simulink model "mrefrobotarm_modified_previous_y_previous_u_previous_ref_prepro"  (R2018b)
settings: Solver=FixedStepAuto  StartTime=0.0  StopTime=10  RelTol=1e-3  AbsTol=1e-6
undefined symbols (not defined in the file or in its folder): cc, options
libraries: neural x594, simulink x1
(part 12 of 22)

== system mrefrobotarm_modified_previous_y_previous_u_previous_ref_prepro/pre_0.00002/Layer 3/Delays 1 ==
  "p{3}" : Inport  PortDimensions=30
      mask Display: e = 0.06;c1 = [120 230 180]/255;c2 = ([120 230 180]+0)/(256+128);c3 = ([120 230 180]+128)/(256+128);patch([0 1 1 0],[0 0 1 1],c1);patch([0 1 1 1-e 1-e 0+e],[0 0 1 1-e 0+e 0+e],c2);patch([0 0 1 1-e 0+e 0+e],[0 1 1 1-e 1-e 0+e],c3);plot([0 1 1 0 0],[0 0 1 1 0]);
  mux : Mux  Inputs=1
      mask Display: e = 0.06;c1 = [120 150 230]/255;c2 = ([120 150 230]+0)/383;c3 = ([120 150 230]+128)/383;patch([0 1 1 0],[0 0 1 1],c1);patch([0 1 1 1-e 1-e 0+e],[0 0 1 1-e 0+e 0+e],c2);patch([0 0 1 1-e 0+e 0+e],[0 1 1 1-e 1-e 0+e],c3);plot([0 1 1 0 0],[0 0 1 1 0]);disp('Mux')
  "pd{3,2}" : Outport
      mask Display: e = 0.06;c1 = [120 230 180]/255;c2 = ([120 230 180]+0)/(256+128);c3 = ([120 230 180]+128)/(256+128);patch([0 1 1 0],[0 0 1 1],c1);patch([0 1 1 1-e 1-e 0+e],[0 0 1 1-e 0+e 0+e],c2);patch([0 0 1 1-e 0+e 0+e],[0 1 1 1-e 1-e 0+e],c3);plot([0 1 1 0 0],[0 0 1 1 0]);
  wires:
  "p{3}"/1 -> mux/1
  mux/1 -> "pd{3,2}"/1

== system mrefrobotarm_modified_previous_y_previous_u_previous_ref_prepro/pre_0.00002/Layer 3/LW{3,2} ==
  "ad{3,2}" : Inport  PortDimensions=30
      mask Display: e = 0.06;c1 = [120 230 180]/255;c2 = ([120 230 180]+0)/(256+128);c3 = ([120 230 180]+128)/(256+128);patch([0 1 1 0],[0 0 1 1],c1);patch([0 1 1 1-e 1-e 0+e],[0 0 1 1-e 0+e 0+e],c2);patch([0 0 1 1-e 0+e 0+e],[0 1 1 1-e 1-e 0+e],c3);plot([0 1 1 0 0],[0 0 1 1 0]);
  "IW{3,2}(1,:)'" : Constant  Value=[0.026357043524044672377915077277066302485764026641845703125;-0.51872721281168232554392716338043101131916046142578125;0.06788526676316682106904210058928583748638629913330078125;0.1504865458343480622005472469027154147624969482421875;0.2009539872745570165957218478069989942014217376708984375;-0.25736048987968518364510828178026713430881500244140625;0.4746746233954628468865166723844595253467559814453125;0.09619380315352972499187700350375962443649768829345703125;-0.39222775076773885860603741093655116856098175048828125;0.58814532203051161918239131409791298210620880126953125;-0.0090835429099451990564428882635183981619775295257568359375;0.02668635591032859910587404783655074425041675567626953125;-0.29710748430544153819710118114016950130462646484375;-0.30678250346949997862111558788456022739410400390625;-0.18096965580139234841539064291282556951045989990234375;-0.65963002624456257283469540197984315454959869384765625;0.483992188838884784818361595171154476702213287353515625;0.0026123351413663013949328917107095548999495804309844970703125;0.02009700292768311358226895890766172669827938079833984375;0.11671148285488382179142519134984468109905719757080078125;-0.134139518384796152528082302524126134812831878662109375;0.34435981653929437218408793341950513422489166259765625;0.151399461664854573239580304289120249450206756591796875;-0.429360650055773229727407169775688089430332183837890625;0.40448496021973412428707206345279701054096221923828125;0.255568865447091175813199015465215779840946197509765625;0.38427145101844495389542544216965325176715850830078125;-0.53491524948961555185888983032782562077045440673828125;0.2358667832365416161533033800878911279141902923583984375;-1.269425035749180974420369238941930234432220458984375]
      mask Display: e = 0.06;c1 = [120 150 230]/255;c2 = ([120 150 230]+0)/383;c3 = ([120 150 230]+128)/383;patch([0 1 1 0],[0 0 1 1],c1);patch([0 1 1 1-e 1-e 0+e],[0 0 1 1-e 0+e 0+e],c2);patch([0 0 1 1-e 0+e 0+e],[0 1 1 1-e 1-e 0+e],c3);plot([0 1 1 0 0],[0 0 1 1 0]);disp('weights');
  Mux : Mux  Inputs=1
      mask Display: e = 0.06;c1 = [120 150 230]/255;c2 = ([120 150 230]+0)/383;c3 = ([120 150 230]+128)/383;patch([0 1 1 0],[0 0 1 1],c1);patch([0 1 1 1-e 1-e 0+e],[0 0 1 1-e 0+e 0+e],c2);patch([0 0 1 1-e 0+e 0+e],[0 1 1 1-e 1-e 0+e],c3);plot([0 1 1 0 0],[0 0 1 1 0]);disp('Mux');
  dotprod1 : neural/Weight Functions/dotprod
  "lz{3,2}" : Outport
      mask Display: e = 0.06;c1 = [120 230 180]/255;c2 = ([120 230 180]+0)/(256+128);c3 = ([120 230 180]+128)/(256+128);patch([0 1 1 0],[0 0 1 1],c1);patch([0 1 1 1-e 1-e 0+e],[0 0 1 1-e 0+e 0+e],c2);patch([0 0 1 1-e 0+e 0+e],[0 1 1 1-e 1-e 0+e],c3);plot([0 1 1 0 0],[0 0 1 1 0]);
  wires:
  "IW{3,2}(1,:)'"/1 -> dotprod1/1
  "ad{3,2}"/1 -> dotprod1/2
  dotprod1/1 -> Mux/1
  Mux/1 -> "lz{3,2}"/1

== system mrefrobotarm_modified_previous_y_previous_u_previous_ref_prepro/pre_0.00003/Layer 1/Delays 1 ==
  "p{1}" : Inport  PortDimensions=10
      mask Display: e = 0.06;c1 = [120 230 180]/255;c2 = ([120 230 180]+0)/(256+128);c3 = ([120 230 180]+128)/(256+128);patch([0 1 1 0],[0 0 1 1],c1);patch([0 1 1 1-e 1-e 0+e],[0 0 1 1-e 0+e 0+e],c2);patch([0 0 1 1-e 0+e 0+e],[0 1 1 1-e 1-e 0+e],c3);plot([0 1 1 0 0],[0 0 1 1 0]);
  mux : Mux  Inputs=1
      mask Display: e = 0.06;c1 = [120 150 230]/255;c2 = ([120 150 230]+0)/383;c3 = ([120 150 230]+128)/383;patch([0 1 1 0],[0 0 1 1],c1);patch([0 1 1 1-e 1-e 0+e],[0 0 1 1-e 0+e 0+e],c2);patch([0 0 1 1-e 0+e 0+e],[0 1 1 1-e 1-e 0+e],c3);plot([0 1 1 0 0],[0 0 1 1 0]);disp('Mux')
  "pd{1,1}" : Outport
      mask Display: e = 0.06;c1 = [120 230 180]/255;c2 = ([120 230 180]+0)/(256+128);c3 = ([120 230 180]+128)/(256+128);patch([0 1 1 0],[0 0 1 1],c1);patch([0 1 1 1-e 1-e 0+e],[0 0 1 1-e 0+e 0+e],c2);patch([0 0 1 1-e 0+e 0+e],[0 1 1 1-e 1-e 0+e],c3);plot([0 1 1 0 0],[0 0 1 1 0]);
  wires:
  "p{1}"/1 -> mux/1
  mux/1 -> "pd{1,1}"/1

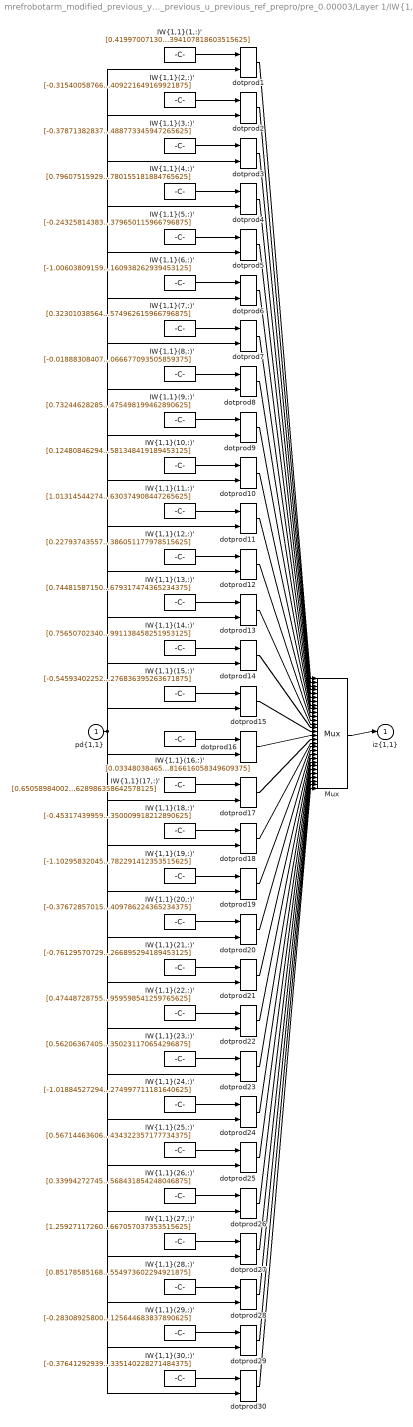
== system mrefrobotarm_modified_previous_y_previous_u_previous_ref_prepro/pre_0.00003/Layer 1/IW{1,1} ==
  "pd{1,1}" : Inport  PortDimensions=10
      mask Display: e = 0.06;c1 = [120 230 180]/255;c2 = ([120 230 180]+0)/(256+128);c3 = ([120 230 180]+128)/(256+128);patch([0 1 1 0],[0 0 1 1],c1);patch([0 1 1 1-e 1-e 0+e],[0 0 1 1-e 0+e 0+e],c2);patch([0 0 1 1-e 0+e 0+e],[0 1 1 1-e 1-e 0+e],c3);plot([0 1 1 0 0],[0 0 1 1 0]);
  "IW{1,1}(1,:)'" : Constant  Value=[0.419970071301938474572779114168952219188213348388671875;-0.8435648108302473691111345033277757465839385986328125;-0.1656764929854205037340619810493080876767635345458984375;-0.11639218277869724238460236165337846614420413970947265625;-1.0085904908462273166236400356865487992763519287109375;0.2870157504733672482188922003842890262603759765625;0.51428228640491180367888546243193559348583221435546875;0.54134778151221329967057727117207832634449005126953125;0.4535298805716763137496627678046934306621551513671875;-0.80929306256536348573860095712007023394107818603515625]
      mask Display: e = 0.06;c1 = [120 150 230]/255;c2 = ([120 150 230]+0)/383;c3 = ([120 150 230]+128)/383;patch([0 1 1 0],[0 0 1 1],c1);patch([0 1 1 1-e 1-e 0+e],[0 0 1 1-e 0+e 0+e],c2);patch([0 0 1 1-e 0+e 0+e],[0 1 1 1-e 1-e 0+e],c3);plot([0 1 1 0 0],[0 0 1 1 0]);disp('Weights');
  "IW{1,1}(10,:)'" : Constant  Value=[0.1248084629473502626950676130945794284343719482421875;0.5561546445854499420846650536986999213695526123046875;-0.000113541552609613440039115772606237442232668399810791015625;-1.267332618187496873218833570717833936214447021484375;1.324848031024380201614576435531489551067352294921875;0.435693687642321469954964641146943904459476470947265625;-0.8716286812435034558887991806841455399990081787109375;0.039256312878930797738430413801324903033673763275146484375;0.24291130218279122221503030232270248234272003173828125;0.579349644472149094553969916887581348419189453125]
      mask Display: e = 0.06;c1 = [120 150 230]/255;c2 = ([120 150 230]+0)/383;c3 = ([120 150 230]+128)/383;patch([0 1 1 0],[0 0 1 1],c1);patch([0 1 1 1-e 1-e 0+e],[0 0 1 1-e 0+e 0+e],c2);patch([0 0 1 1-e 0+e 0+e],[0 1 1 1-e 1-e 0+e],c3);plot([0 1 1 0 0],[0 0 1 1 0]);disp('Weights');
  "IW{1,1}(11,:)'" : Constant  Value=[1.013145442746719471216465535690076649188995361328125;0.99243177005728810957663199587841518223285675048828125;0.7891671128990978001382927686790935695171356201171875;0.99448519338468754913407110507250763475894927978515625;0.78513301503203092313043498506885953247547149658203125;1.039734908888301223583994215005077421665191650390625;0.0113187088607663612072062875313349650241434574127197265625;0.450506637373380869338035381588269956409931182861328125;0.463038284909750241791215330522391013801097869873046875;0.08865900952312423533019369870089576579630374908447265625]
      mask Display: e = 0.06;c1 = [120 150 230]/255;c2 = ([120 150 230]+0)/383;c3 = ([120 150 230]+128)/383;patch([0 1 1 0],[0 0 1 1],c1);patch([0 1 1 1-e 1-e 0+e],[0 0 1 1-e 0+e 0+e],c2);patch([0 0 1 1-e 0+e 0+e],[0 1 1 1-e 1-e 0+e],c3);plot([0 1 1 0 0],[0 0 1 1 0]);disp('Weights');
  "IW{1,1}(12,:)'" : Constant  Value=[0.2279374355718996325581571227303356863558292388916015625;-0.72859698297398123312262896433821879327297210693359375;0.47417467679467184549224612055695615708827972412109375;0.990640763171337201953292606049217283725738525390625;0.09802646157368609391991043366942903958261013031005859375;-0.1375834764035423207761965613826760090887546539306640625;0.94485525986767082695649833112838678061962127685546875;-0.089139203371477238047049240776686929166316986083984375;0.348785768332843748584792820111033506691455841064453125;-0.70331874474973388178256072933436371386051177978515625]
      mask Display: e = 0.06;c1 = [120 150 230]/255;c2 = ([120 150 230]+0)/383;c3 = ([120 150 230]+128)/383;patch([0 1 1 0],[0 0 1 1],c1);patch([0 1 1 1-e 1-e 0+e],[0 0 1 1-e 0+e 0+e],c2);patch([0 0 1 1-e 0+e 0+e],[0 1 1 1-e 1-e 0+e],c3);plot([0 1 1 0 0],[0 0 1 1 0]);disp('Weights');
  "IW{1,1}(13,:)'" : Constant  Value=[0.7448158715080184233414684058516286313533782958984375;-0.937709653184260805147687278804369270801544189453125;0.21308729556658556614223698488785885274410247802734375;0.89987770978577519276342400189605541527271270751953125;-0.5439743765683768828012034646235406398773193359375;1.540566291152452915724779813899658620357513427734375;-0.1376689897811968210650235278080799616873264312744140625;-0.228351277546065489776339063610066659748554229736328125;0.038462164544626441242680670029585598967969417572021484375;-0.57219919711055788891229667569859884679317474365234375]
      mask Display: e = 0.06;c1 = [120 150 230]/255;c2 = ([120 150 230]+0)/383;c3 = ([120 150 230]+128)/383;patch([0 1 1 0],[0 0 1 1],c1);patch([0 1 1 1-e 1-e 0+e],[0 0 1 1-e 0+e 0+e],c2);patch([0 0 1 1-e 0+e 0+e],[0 1 1 1-e 1-e 0+e],c3);plot([0 1 1 0 0],[0 0 1 1 0]);disp('Weights');
  "IW{1,1}(14,:)'" : Constant  Value=[0.7565070234021742390240206077578477561473846435546875;-0.2269197034980003080395505321575910784304141998291015625;0.027723441230358518427845382348095881752669811248779296875;0.391467362700477272685617435854510404169559478759765625;0.54147453576161541644040653409319929778575897216796875;0.782900867393638844049519320833496749401092529296875;-0.00425243933368514397119763970067651825957000255584716796875;-1.1264556989739828996022197316051460802555084228515625;-0.394415400911664548733170931882341392338275909423828125;0.559938589090539284853775825467891991138458251953125]
      mask Display: e = 0.06;c1 = [120 150 230]/255;c2 = ([120 150 230]+0)/383;c3 = ([120 150 230]+128)/383;patch([0 1 1 0],[0 0 1 1],c1);patch([0 1 1 1-e 1-e 0+e],[0 0 1 1-e 0+e 0+e],c2);patch([0 0 1 1-e 0+e 0+e],[0 1 1 1-e 1-e 0+e],c3);plot([0 1 1 0 0],[0 0 1 1 0]);disp('Weights');
  "IW{1,1}(15,:)'" : Constant  Value=[-0.5459340225233961785278324896353296935558319091796875;1.0013274219639980433527171044261194765567779541015625;-0.10478805573236359138800111168166040442883968353271484375;-0.39791550833071187565082027504104189574718475341796875;-1.8226347375210345536089562301640398800373077392578125;1.1549295657493761080303329435992054641246795654296875;-0.44044889877680348799771081758080981671810150146484375;0.62148745105600744498275389560149051249027252197265625;-1.02846840266751815562429328565485775470733642578125;-0.36827462238854991039005426500807516276836395263671875]
      mask Display: e = 0.06;c1 = [120 150 230]/255;c2 = ([120 150 230]+0)/383;c3 = ([120 150 230]+128)/383;patch([0 1 1 0],[0 0 1 1],c1);patch([0 1 1 1-e 1-e 0+e],[0 0 1 1-e 0+e 0+e],c2);patch([0 0 1 1-e 0+e 0+e],[0 1 1 1-e 1-e 0+e],c3);plot([0 1 1 0 0],[0 0 1 1 0]);disp('Weights');
  "IW{1,1}(16,:)'" : Constant  Value=[0.03348038465723013334951474462286569178104400634765625;-0.75171930775220208165166013714042492210865020751953125;-1.0015168648609507062730017423746176064014434814453125;-0.61533840092821223688446252708672545850276947021484375;1.0940863389095272228956901017227210104465484619140625;0.40757548665249598851545442812494002282619476318359375;0.10340982664735391682864218410031753592193126678466796875;-0.113628985649216363018609854407259263098239898681640625;-1.0602476694165130499669658092898316681385040283203125;-0.2049179980871381479001769321257597766816616058349609375]
      mask Display: e = 0.06;c1 = [120 150 230]/255;c2 = ([120 150 230]+0)/383;c3 = ([120 150 230]+128)/383;patch([0 1 1 0],[0 0 1 1],c1);patch([0 1 1 1-e 1-e 0+e],[0 0 1 1-e 0+e 0+e],c2);patch([0 0 1 1-e 0+e 0+e],[0 1 1 1-e 1-e 0+e],c3);plot([0 1 1 0 0],[0 0 1 1 0]);disp('Weights');
  "IW{1,1}(17,:)'" : Constant  Value=[0.650589840024939913831758531159721314907073974609375;-0.61786799583753337916647296879091300070285797119140625;0.63821081218878694674145890530780889093875885009765625;-0.28877908003107621848215558202355168759822845458984375;0.339548676092817081073604867924586869776248931884765625;-0.05333696531103850058119775212617241777479648590087890625;-0.97890616367028171485031862175674177706241607666015625;0.54470130680517614418789662522613070905208587646484375;-0.77061417573863055796579146772273816168308258056640625;-0.71305265072652368463224092920427210628986358642578125]
      mask Display: e = 0.06;c1 = [120 150 230]/255;c2 = ([120 150 230]+0)/383;c3 = ([120 150 230]+128)/383;patch([0 1 1 0],[0 0 1 1],c1);patch([0 1 1 1-e 1-e 0+e],[0 0 1 1-e 0+e 0+e],c2);patch([0 0 1 1-e 0+e 0+e],[0 1 1 1-e 1-e 0+e],c3);plot([0 1 1 0 0],[0 0 1 1 0]);disp('Weights');
  "IW{1,1}(18,:)'" : Constant  Value=[-0.45317439959418237549471086822450160980224609375;1.012172744591367301580930870841257274150848388671875;0.7505435143556933308417455918970517814159393310546875;0.99313324530325852723677826361381448805332183837890625;-0.173991191613037832208732424987829290330410003662109375;1.0131996572588637395284649755922146141529083251953125;0.325960642115960042008993013951112516224384307861328125;-0.483341987178338816644185271798050962388515472412109375;0.0173491836073219295177860743706332868896424770355224609375;-0.57800826004801886259798493483685888350009918212890625]
      mask Display: e = 0.06;c1 = [120 150 230]/255;c2 = ([120 150 230]+0)/383;c3 = ([120 150 230]+128)/383;patch([0 1 1 0],[0 0 1 1],c1);patch([0 1 1 1-e 1-e 0+e],[0 0 1 1-e 0+e 0+e],c2);patch([0 0 1 1-e 0+e 0+e],[0 1 1 1-e 1-e 0+e],c3);plot([0 1 1 0 0],[0 0 1 1 0]);disp('Weights');
  "IW{1,1}(19,:)'" : Constant  Value=[-1.1029583204535384766131755895912647247314453125;0.0867889546048641047359950562167796306312084197998046875;0.20130105959816602112510963706881739199161529541015625;-0.03269779935203391552089868810071493498980998992919921875;-0.809986526790105632045424499665386974811553955078125;-0.9940615751205121863876001953030936419963836669921875;-0.449578022569887936210619727717130444943904876708984375;1.292200048466627837484566043713130056858062744140625;0.1583121664471566492071730181123712100088596343994140625;0.06975499456212576332436725579100311733782291412353515625]
      mask Display: e = 0.06;c1 = [120 150 230]/255;c2 = ([120 150 230]+0)/383;c3 = ([120 150 230]+128)/383;patch([0 1 1 0],[0 0 1 1],c1);patch([0 1 1 1-e 1-e 0+e],[0 0 1 1-e 0+e 0+e],c2);patch([0 0 1 1-e 0+e 0+e],[0 1 1 1-e 1-e 0+e],c3);plot([0 1 1 0 0],[0 0 1 1 0]);disp('Weights');
  "IW{1,1}(2,:)'" : Constant  Value=[-0.315400587669002419044517182555864565074443817138671875;1.2154371235917660332148670931928791105747222900390625;-0.83423375061050097922787927018362097442150115966796875;0.3787632570847225821353276842273771762847900390625;0.5752622342607571770400909372256137430667877197265625;-0.9461684407448653910677194289746694266796112060546875;0.57910774236140394322092106449417769908905029296875;-0.08803539023674993024837220900735701434314250946044921875;-0.11631975131734097195224109100308851338922977447509765625;-0.039099357899579682829038773661523009650409221649169921875]
      mask Display: e = 0.06;c1 = [120 150 230]/255;c2 = ([120 150 230]+0)/383;c3 = ([120 150 230]+128)/383;patch([0 1 1 0],[0 0 1 1],c1);patch([0 1 1 1-e 1-e 0+e],[0 0 1 1-e 0+e 0+e],c2);patch([0 0 1 1-e 0+e 0+e],[0 1 1 1-e 1-e 0+e],c3);plot([0 1 1 0 0],[0 0 1 1 0]);disp('Weights');
  "IW{1,1}(20,:)'" : Constant  Value=[-0.3767285701595624036741583040566183626651763916015625;0.0926343571210796745685200903608347289264202117919921875;-0.397908041895699449153056548311724327504634857177734375;0.0911491372255521792311583340051583945751190185546875;-0.521535930069929154484498212696053087711334228515625;1.6981905001688806233772766063339076936244964599609375;-0.7031228568751888285959239510702900588512420654296875;-0.16942067461137588768593786880956031382083892822265625;1.011359321001015221241914332495070993900299072265625;0.2292475188820937981315495335365994833409786224365234375]
      mask Display: e = 0.06;c1 = [120 150 230]/255;c2 = ([120 150 230]+0)/383;c3 = ([120 150 230]+128)/383;patch([0 1 1 0],[0 0 1 1],c1);patch([0 1 1 1-e 1-e 0+e],[0 0 1 1-e 0+e 0+e],c2);patch([0 0 1 1-e 0+e 0+e],[0 1 1 1-e 1-e 0+e],c3);plot([0 1 1 0 0],[0 0 1 1 0]);disp('Weights');
  "IW{1,1}(21,:)'" : Constant  Value=[-0.76129570729234374848459765416919253766536712646484375;-0.1865165687287015094941722281873808242380619049072265625;-0.428419790601098415816494480168330483138561248779296875;-0.64711956925728408851483663966064341366291046142578125;1.235955092770737007157322295824997127056121826171875;0.96312903397833060648025593764032237231731414794921875;-1.4627378968582291918210103176534175872802734375;-0.9744466401862297288971603848040103912353515625;-0.384115693737802355034460788374417461454868316650390625;0.65949368504693683945561133441515266895294189453125]
      mask Display: e = 0.06;c1 = [120 150 230]/255;c2 = ([120 150 230]+0)/383;c3 = ([120 150 230]+128)/383;patch([0 1 1 0],[0 0 1 1],c1);patch([0 1 1 1-e 1-e 0+e],[0 0 1 1-e 0+e 0+e],c2);patch([0 0 1 1-e 0+e 0+e],[0 1 1 1-e 1-e 0+e],c3);plot([0 1 1 0 0],[0 0 1 1 0]);disp('Weights');
  "IW{1,1}(22,:)'" : Constant  Value=[0.474487287550881042808015308764879591763019561767578125;-0.523872412146371591035176606965251266956329345703125;0.271121607040405054878107193871983326971530914306640625;0.5311413832030760229230281765921972692012786865234375;-0.54191421303600595393845651415176689624786376953125;-0.76999759614602714119513393598026596009731292724609375;1.192167804042037371203832663013599812984466552734375;0.370831219659940980459822412740322761237621307373046875;0.67306378875913275283693337769364006817340850830078125;0.71638288814274508897739224266842938959598541259765625]
      mask Display: e = 0.06;c1 = [120 150 230]/255;c2 = ([120 150 230]+0)/383;c3 = ([120 150 230]+128)/383;patch([0 1 1 0],[0 0 1 1],c1);patch([0 1 1 1-e 1-e 0+e],[0 0 1 1-e 0+e 0+e],c2);patch([0 0 1 1-e 0+e 0+e],[0 1 1 1-e 1-e 0+e],c3);plot([0 1 1 0 0],[0 0 1 1 0]);disp('Weights');
  "IW{1,1}(23,:)'" : Constant  Value=[0.5620636740579298962217080770642496645450592041015625;0.354753702489910505146752939253929071128368377685546875;0.334857219881603274114212354106712155044078826904296875;-0.68939539769561586357582427808665670454502105712890625;0.352851915411073469019953563474700786173343658447265625;1.1447344029547517063605255316360853612422943115234375;-1.03579785054005046873726314515806734561920166015625;-0.7021063634165380928919830694212578237056732177734375;-0.398210344971560326055026735048159025609493255615234375;-0.25210744532015272323377530483412556350231170654296875]
      mask Display: e = 0.06;c1 = [120 150 230]/255;c2 = ([120 150 230]+0)/383;c3 = ([120 150 230]+128)/383;patch([0 1 1 0],[0 0 1 1],c1);patch([0 1 1 1-e 1-e 0+e],[0 0 1 1-e 0+e 0+e],c2);patch([0 0 1 1-e 0+e 0+e],[0 1 1 1-e 1-e 0+e],c3);plot([0 1 1 0 0],[0 0 1 1 0]);disp('Weights');
  "IW{1,1}(24,:)'" : Constant  Value=[-1.018845272944447710727899902849458158016204833984375;0.491836262087783637753091170452535152435302734375;0.75512179162889514483225639196461997926235198974609375;-0.2527361397636418427481430626357905566692352294921875;1.2325799684120966048794798552989959716796875;-0.63349017733743984148730987726594321429729461669921875;-0.27389861630554956928307319685700349509716033935546875;-0.39648248008667186237374835400260053575038909912109375;-0.257740972322303918407015999036957509815692901611328125;0.417434105134619815036245427108951844274997711181640625]
      mask Display: e = 0.06;c1 = [120 150 230]/255;c2 = ([120 150 230]+0)/383;c3 = ([120 150 230]+128)/383;patch([0 1 1 0],[0 0 1 1],c1);patch([0 1 1 1-e 1-e 0+e],[0 0 1 1-e 0+e 0+e],c2);patch([0 0 1 1-e 0+e 0+e],[0 1 1 1-e 1-e 0+e],c3);plot([0 1 1 0 0],[0 0 1 1 0]);disp('Weights');
  "IW{1,1}(25,:)'" : Constant  Value=[0.5671446360696845712112690307549200952053070068359375;-0.5304720897289534331520144405658356845378875732421875;-0.77524781661523689546555715423892252147197723388671875;-0.0922370551799614191157417053545941598713397979736328125;1.188743973357082150954511234886012971401214599609375;-0.7349542103368633672033638504217378795146942138671875;-0.4218373955702710009774136779014952480792999267578125;-0.73691835737733957234496529054013080894947052001953125;0.04489836297479889160033650341574684716761112213134765625;-0.8440497817406418246122257187380455434322357177734375]
      mask Display: e = 0.06;c1 = [120 150 230]/255;c2 = ([120 150 230]+0)/383;c3 = ([120 150 230]+128)/383;patch([0 1 1 0],[0 0 1 1],c1);patch([0 1 1 1-e 1-e 0+e],[0 0 1 1-e 0+e 0+e],c2);patch([0 0 1 1-e 0+e 0+e],[0 1 1 1-e 1-e 0+e],c3);plot([0 1 1 0 0],[0 0 1 1 0]);disp('Weights');
  "IW{1,1}(26,:)'" : Constant  Value=[0.339942727454486448568360401623067446053028106689453125;-0.498638976556827928643400582586764357984066009521484375;-0.07295796636774475041331555758006288670003414154052734375;0.8865373711675250678609927490469999611377716064453125;-0.689393309727687420007669061305932700634002685546875;0.32558781113365220516442377629573456943035125732421875;0.66995933247233419027821810232126154005527496337890625;0.93757848559566314694535549278953112661838531494140625;-0.427062855211565395308070947066880762577056884765625;-0.39322691891576677658548533145221881568431854248046875]
      mask Display: e = 0.06;c1 = [120 150 230]/255;c2 = ([120 150 230]+0)/383;c3 = ([120 150 230]+128)/383;patch([0 1 1 0],[0 0 1 1],c1);patch([0 1 1 1-e 1-e 0+e],[0 0 1 1-e 0+e 0+e],c2);patch([0 0 1 1-e 0+e 0+e],[0 1 1 1-e 1-e 0+e],c3);plot([0 1 1 0 0],[0 0 1 1 0]);disp('Weights');
  "IW{1,1}(27,:)'" : Constant  Value=[1.2592711726058276600070939821307547390460968017578125;0.64224385925763005644739678245969116687774658203125;-0.53474192921636698461185233099968172609806060791015625;-0.59978461662693705047644243677495978772640228271484375;0.34923896027142287135092146854731254279613494873046875;-0.290141567064720662383336957645951770246028900146484375;0.1913235471734429093970675239688716828823089599609375;-1.0193921480099905618743605373310856521129608154296875;-0.31385910713233367008712093593203462660312652587890625;-0.2166281288631170254266322672265232540667057037353515625]
      mask Display: e = 0.06;c1 = [120 150 230]/255;c2 = ([120 150 230]+0)/383;c3 = ([120 150 230]+128)/383;patch([0 1 1 0],[0 0 1 1],c1);patch([0 1 1 1-e 1-e 0+e],[0 0 1 1-e 0+e 0+e],c2);patch([0 0 1 1-e 0+e 0+e],[0 1 1 1-e 1-e 0+e],c3);plot([0 1 1 0 0],[0 0 1 1 0]);disp('Weights');
  "IW{1,1}(28,:)'" : Constant  Value=[0.85178585168483766931757372731226496398448944091796875;0.97939739620257537655589885616791434586048126220703125;-0.0559270363052022656535910982711357064545154571533203125;-0.645607784756814684357095757150091230869293212890625;-0.04681377542786428758159189555954071693122386932373046875;-0.13749018353687814109065357115468941628932952880859375;-0.1792414174404352300573606271427706815302371978759765625;-0.78099786999265929932079188802163116633892059326171875;-0.71601537465538223070637968703522346913814544677734375;0.00724674116364962088432388753744817222468554973602294921875]
      mask Display: e = 0.06;c1 = [120 150 230]/255;c2 = ([120 150 230]+0)/383;c3 = ([120 150 230]+128)/383;patch([0 1 1 0],[0 0 1 1],c1);patch([0 1 1 1-e 1-e 0+e],[0 0 1 1-e 0+e 0+e],c2);patch([0 0 1 1-e 0+e 0+e],[0 1 1 1-e 1-e 0+e],c3);plot([0 1 1 0 0],[0 0 1 1 0]);disp('Weights');
  "IW{1,1}(29,:)'" : Constant  Value=[-0.2830892580084742871093794747139327228069305419921875;-0.73242541957172180300261743468581698834896087646484375;-0.51591206743478668084179616926121525466442108154296875;1.0349976588705658286926336586475372314453125;-0.08941806714276907819272111055397544987499713897705078125;-0.28418816470434637988518034035223536193370819091796875;0.519810505523996990717705557472072541713714599609375;-0.83450384569327329398191750442492775619029998779296875;-0.84401513729662280827170661723357625305652618408203125;-0.038381954797233365506148317081169807352125644683837890625]
      mask Display: e = 0.06;c1 = [120 150 230]/255;c2 = ([120 150 230]+0)/383;c3 = ([120 150 230]+128)/383;patch([0 1 1 0],[0 0 1 1],c1);patch([0 1 1 1-e 1-e 0+e],[0 0 1 1-e 0+e 0+e],c2);patch([0 0 1 1-e 0+e 0+e],[0 1 1 1-e 1-e 0+e],c3);plot([0 1 1 0 0],[0 0 1 1 0]);disp('Weights');
  "IW{1,1}(3,:)'" : Constant  Value=[-0.3787138283723165965710677483002655208110809326171875;0.483982128419606583147327683036564849317073822021484375;0.406763930229814552053113629881408996880054473876953125;0.96390052727149166944542457713396288454532623291015625;-0.5563925325548273459475012714392505586147308349609375;0.418750045839037243755598183270194567739963531494140625;-0.350668822228053567169325788199785165488719940185546875;0.440431914235321908535070178913883864879608154296875;1.1067064669781512264989942195825278759002685546875;0.36184998074264262957200344317243434488773345947265625]
      mask Display: e = 0.06;c1 = [120 150 230]/255;c2 = ([120 150 230]+0)/383;c3 = ([120 150 230]+128)/383;patch([0 1 1 0],[0 0 1 1],c1);patch([0 1 1 1-e 1-e 0+e],[0 0 1 1-e 0+e 0+e],c2);patch([0 0 1 1-e 0+e 0+e],[0 1 1 1-e 1-e 0+e],c3);plot([0 1 1 0 0],[0 0 1 1 0]);disp('Weights');
  "IW{1,1}(30,:)'" : Constant  Value=[-0.376412929391506001497447186920908279716968536376953125;-0.23793748056435981563794257453992031514644622802734375;0.70051350580105509191497503707068972289562225341796875;0.1760620440330393499106520494024152867496013641357421875;0.6858422814878768480895132597652263939380645751953125;0.206916515454207028401611978551954962313175201416015625;0.75379028220662558368303507450036704540252685546875;0.44452107543207597384338214396848343312740325927734375;1.029760748722175822678082113270647823810577392578125;0.459555350335039081155485973795293830335140228271484375]
      mask Display: e = 0.06;c1 = [120 150 230]/255;c2 = ([120 150 230]+0)/383;c3 = ([120 150 230]+128)/383;patch([0 1 1 0],[0 0 1 1],c1);patch([0 1 1 1-e 1-e 0+e],[0 0 1 1-e 0+e 0+e],c2);patch([0 0 1 1-e 0+e 0+e],[0 1 1 1-e 1-e 0+e],c3);plot([0 1 1 0 0],[0 0 1 1 0]);disp('Weights');
  "IW{1,1}(4,:)'" : Constant  Value=[0.79607515929074423866040888242423534393310546875;-0.3506933710821911187593968861619941890239715576171875;0.055750784674063739998484123816524515859782695770263671875;0.68339674823100027278854895484982989728450775146484375;-1.1321930481874187268687137475353665649890899658203125;1.5135919981996881489294537459500133991241455078125;0.24913388805575908957479214222985319793224334716796875;-0.195788956514948819798149770576856099069118499755859375;-0.35746860668333735322477195950341410934925079345703125;-0.52852126326601567285479177371598780155181884765625]
      mask Display: e = 0.06;c1 = [120 150 230]/255;c2 = ([120 150 230]+0)/383;c3 = ([120 150 230]+128)/383;patch([0 1 1 0],[0 0 1 1],c1);patch([0 1 1 1-e 1-e 0+e],[0 0 1 1-e 0+e 0+e],c2);patch([0 0 1 1-e 0+e 0+e],[0 1 1 1-e 1-e 0+e],c3);plot([0 1 1 0 0],[0 0 1 1 0]);disp('Weights');
  "IW{1,1}(5,:)'" : Constant  Value=[-0.2432581438341555879478761426071287132799625396728515625;0.64905369984275773642679041586234234273433685302734375;-0.292710795883404373274316867536981590092182159423828125;0.64531406673956703823336056302650831639766693115234375;-0.322941665561168156362015224658534862101078033447265625;0.78603355615901981945370380344684235751628875732421875;0.84156401662527036133809588136500678956508636474609375;0.334050987477957084248458841102547012269496917724609375;0.1693903489510988347177544710575602948665618896484375;-0.895946407747902906493209229665808379650115966796875]
      mask Display: e = 0.06;c1 = [120 150 230]/255;c2 = ([120 150 230]+0)/383;c3 = ([120 150 230]+128)/383;patch([0 1 1 0],[0 0 1 1],c1);patch([0 1 1 1-e 1-e 0+e],[0 0 1 1-e 0+e 0+e],c2);patch([0 0 1 1-e 0+e 0+e],[0 1 1 1-e 1-e 0+e],c3);plot([0 1 1 0 0],[0 0 1 1 0]);disp('Weights');
  "IW{1,1}(6,:)'" : Constant  Value=[-1.00603809159993407007505084038712084293365478515625;-0.482841889231014176342426935661933384835720062255859375;-0.66525803998977572906170507849310524761676788330078125;-0.99752027269883580817833035325747914612293243408203125;-0.695296951396717322069207511958666145801544189453125;-0.9334827838031143354413643464795313775539398193359375;0.00504539256601603015861545742382077150978147983551025390625;-0.92491698242550957065333250284311361610889434814453125;0.76087420108080194847133270741323940455913543701171875;0.1792929048685512061211966283735819160938262939453125]
      mask Display: e = 0.06;c1 = [120 150 230]/255;c2 = ([120 150 230]+0)/383;c3 = ([120 150 230]+128)/383;patch([0 1 1 0],[0 0 1 1],c1);patch([0 1 1 1-e 1-e 0+e],[0 0 1 1-e 0+e 0+e],c2);patch([0 0 1 1-e 0+e 0+e],[0 1 1 1-e 1-e 0+e],c3);plot([0 1 1 0 0],[0 0 1 1 0]);disp('Weights');
  "IW{1,1}(7,:)'" : Constant  Value=[0.323010385647662323638229509015218354761600494384765625;0.7459260735533141950526214714045636355876922607421875;-0.79517242151492173451998723976430483162403106689453125;0.59309679654623492783827032326371408998966217041015625;0.2202193407666629132446445282766944728791713714599609375;-0.455108161436382163689273738782503642141819000244140625;0.96976334619942983206186681854887865483760833740234375;-0.10878851600937687604808701280489913187921047210693359375;-0.0542308313305440992113659604001441039144992828369140625;0.60536034128806892606888823138433508574962615966796875]
      mask Display: e = 0.06;c1 = [120 150 230]/255;c2 = ([120 150 230]+0)/383;c3 = ([120 150 230]+128)/383;patch([0 1 1 0],[0 0 1 1],c1);patch([0 1 1 1-e 1-e 0+e],[0 0 1 1-e 0+e 0+e],c2);patch([0 0 1 1-e 0+e 0+e],[0 1 1 1-e 1-e 0+e],c3);plot([0 1 1 0 0],[0 0 1 1 0]);disp('Weights');
  "IW{1,1}(8,:)'" : Constant  Value=[-0.0188830840791791854105241554862004704773426055908203125;0.52841526198398269809075600278447382152080535888671875;-0.7636736677294351238742819987237453460693359375;0.1872688219556681576971612912529963068664073944091796875;0.9797553781840202535846628961735405027866363525390625;-0.688991725608501415223372532636858522891998291015625;0.701371220255219807171442880644463002681732177734375;-0.38854784244459350528444474548450671136379241943359375;0.61071536187409913853940679473453201353549957275390625;0.277945728666647295934666317407391034066677093505859375]
      mask Display: e = 0.06;c1 = [120 150 230]/255;c2 = ([120 150 230]+0)/383;c3 = ([120 150 230]+128)/383;patch([0 1 1 0],[0 0 1 1],c1);patch([0 1 1 1-e 1-e 0+e],[0 0 1 1-e 0+e 0+e],c2);patch([0 0 1 1-e 0+e 0+e],[0 1 1 1-e 1-e 0+e],c3);plot([0 1 1 0 0],[0 0 1 1 0]);disp('Weights');
  "IW{1,1}(9,:)'" : Constant  Value=[0.73244628285490975816429681799490936100482940673828125;-1.086646870390212793466844232170842587947845458984375;0.519849200721463677865585850668139755725860595703125;-0.1460378358329177117536090690919081680476665496826171875;-0.323124687307321190044007153119309805333614349365234375;0.64896490844555809740512586358818225562572479248046875;-0.4930543043532702451869909054948948323726654052734375;0.118113734372571166364451755725895054638385772705078125;0.07802985035500442645428620380698703229427337646484375;0.6934318685771254653360529118799604475498199462890625]
      mask Display: e = 0.06;c1 = [120 150 230]/255;c2 = ([120 150 230]+0)/383;c3 = ([120 150 230]+128)/383;patch([0 1 1 0],[0 0 1 1],c1);patch([0 1 1 1-e 1-e 0+e],[0 0 1 1-e 0+e 0+e],c2);patch([0 0 1 1-e 0+e 0+e],[0 1 1 1-e 1-e 0+e],c3);plot([0 1 1 0 0],[0 0 1 1 0]);disp('Weights');
  Mux : Mux  Inputs=30
      mask Display: e = 0.06;c1 = [120 150 230]/255;c2 = ([120 150 230]+0)/383;c3 = ([120 150 230]+128)/383;patch([0 1 1 0],[0 0 1 1],c1);patch([0 1 1 1-e 1-e 0+e],[0 0 1 1-e 0+e 0+e],c2);patch([0 0 1 1-e 0+e 0+e],[0 1 1 1-e 1-e 0+e],c3);plot([0 1 1 0 0],[0 0 1 1 0]);disp('Mux');
  dotprod{1..30} (30 alike) : neural/Weight Functions/dotprod
  "iz{1,1}" : Outport
      mask Display: e = 0.06;c1 = [120 230 180]/255;c2 = ([120 230 180]+0)/(256+128);c3 = ([120 230 180]+128)/(256+128);patch([0 1 1 0],[0 0 1 1],c1);patch([0 1 1 1-e 1-e 0+e],[0 0 1 1-e 0+e 0+e],c2);patch([0 0 1 1-e 0+e 0+e],[0 1 1 1-e 1-e 0+e],c3);plot([0 1 1 0 0],[0 0 1 1 0]);
  wires:
  "IW{1,1}(1,:)'"/1 -> dotprod1/1
  "pd{1,1}"/1 -> dotprod1/2, dotprod2/2, dotprod3/2, dotprod4/2, dotprod5/2, dotprod6/2, dotprod7/2, dotprod8/2, dotprod9/2, dotprod10/2, dotprod11/2, dotprod12/2, dotprod13/2, dotprod14/2, dotprod15/2, dotprod16/2, dotprod17/2, dotprod18/2, dotprod19/2, dotprod20/2, dotprod21/2, dotprod22/2, dotprod23/2, dotprod24/2, dotprod25/2, dotprod26/2, dotprod27/2, dotprod28/2, dotprod29/2, dotprod30/2
  dotprod1/1 -> Mux/1
  "IW{1,1}(2,:)'"/1 -> dotprod2/1
  dotprod2/1 -> Mux/2
  "IW{1,1}(3,:)'"/1 -> dotprod3/1
  dotprod3/1 -> Mux/3
  "IW{1,1}(4,:)'"/1 -> dotprod4/1
  dotprod4/1 -> Mux/4
  "IW{1,1}(5,:)'"/1 -> dotprod5/1
  dotprod5/1 -> Mux/5
  "IW{1,1}(6,:)'"/1 -> dotprod6/1
  dotprod6/1 -> Mux/6
  "IW{1,1}(7,:)'"/1 -> dotprod7/1
  dotprod7/1 -> Mux/7
  "IW{1,1}(8,:)'"/1 -> dotprod8/1
  dotprod8/1 -> Mux/8
  "IW{1,1}(9,:)'"/1 -> dotprod9/1
  dotprod9/1 -> Mux/9
  "IW{1,1}(10,:)'"/1 -> dotprod10/1
  dotprod10/1 -> Mux/10
  "IW{1,1}(11,:)'"/1 -> dotprod11/1
  dotprod11/1 -> Mux/11
  "IW{1,1}(12,:)'"/1 -> dotprod12/1
  dotprod12/1 -> Mux/12
  "IW{1,1}(13,:)'"/1 -> dotprod13/1
  dotprod13/1 -> Mux/13
  "IW{1,1}(14,:)'"/1 -> dotprod14/1
  dotprod14/1 -> Mux/14
  "IW{1,1}(15,:)'"/1 -> dotprod15/1
  dotprod15/1 -> Mux/15
  "IW{1,1}(16,:)'"/1 -> dotprod16/1
  dotprod16/1 -> Mux/16
  "IW{1,1}(17,:)'"/1 -> dotprod17/1
  dotprod17/1 -> Mux/17
  "IW{1,1}(18,:)'"/1 -> dotprod18/1
  dotprod18/1 -> Mux/18
  "IW{1,1}(19,:)'"/1 -> dotprod19/1
  dotprod19/1 -> Mux/19
  "IW{1,1}(20,:)'"/1 -> dotprod20/1
  dotprod20/1 -> Mux/20
  "IW{1,1}(21,:)'"/1 -> dotprod21/1
  dotprod21/1 -> Mux/21
  "IW{1,1}(22,:)'"/1 -> dotprod22/1
  dotprod22/1 -> Mux/22
  "IW{1,1}(23,:)'"/1 -> dotprod23/1
  dotprod23/1 -> Mux/23
  "IW{1,1}(24,:)'"/1 -> dotprod24/1
  dotprod24/1 -> Mux/24
  "IW{1,1}(25,:)'"/1 -> dotprod25/1
  dotprod25/1 -> Mux/25
  "IW{1,1}(26,:)'"/1 -> dotprod26/1
  dotprod26/1 -> Mux/26
  "IW{1,1}(27,:)'"/1 -> dotprod27/1
  dotprod27/1 -> Mux/27
  "IW{1,1}(28,:)'"/1 -> dotprod28/1
  dotprod28/1 -> Mux/28
  "IW{1,1}(29,:)'"/1 -> dotprod29/1
  dotprod29/1 -> Mux/29
  "IW{1,1}(30,:)'"/1 -> dotprod30/1
  dotprod30/1 -> Mux/30
  Mux/1 -> "iz{1,1}"/1

== system mrefrobotarm_modified_previous_y_previous_u_previous_ref_prepro/pre_0.00003/Layer 2/Delays 1 ==
  "p{2}" : Inport  PortDimensions=30
      mask Display: e = 0.06;c1 = [120 230 180]/255;c2 = ([120 230 180]+0)/(256+128);c3 = ([120 230 180]+128)/(256+128);patch([0 1 1 0],[0 0 1 1],c1);patch([0 1 1 1-e 1-e 0+e],[0 0 1 1-e 0+e 0+e],c2);patch([0 0 1 1-e 0+e 0+e],[0 1 1 1-e 1-e 0+e],c3);plot([0 1 1 0 0],[0 0 1 1 0]);
  mux : Mux  Inputs=1
      mask Display: e = 0.06;c1 = [120 150 230]/255;c2 = ([120 150 230]+0)/383;c3 = ([120 150 230]+128)/383;patch([0 1 1 0],[0 0 1 1],c1);patch([0 1 1 1-e 1-e 0+e],[0 0 1 1-e 0+e 0+e],c2);patch([0 0 1 1-e 0+e 0+e],[0 1 1 1-e 1-e 0+e],c3);plot([0 1 1 0 0],[0 0 1 1 0]);disp('Mux')
  "pd{2,1}" : Outport
      mask Display: e = 0.06;c1 = [120 230 180]/255;c2 = ([120 230 180]+0)/(256+128);c3 = ([120 230 180]+128)/(256+128);patch([0 1 1 0],[0 0 1 1],c1);patch([0 1 1 1-e 1-e 0+e],[0 0 1 1-e 0+e 0+e],c2);patch([0 0 1 1-e 0+e 0+e],[0 1 1 1-e 1-e 0+e],c3);plot([0 1 1 0 0],[0 0 1 1 0]);
  wires:
  "p{2}"/1 -> mux/1
  mux/1 -> "pd{2,1}"/1
